simulink model "transfer_function_question_4_closed_loop"  (R2023b)
settings: Solver=VariableStepAuto  StartTime=0.0  StopTime=40  RelTol=1e-3
settings Model: Creator=orife  LastModifiedBy=orife

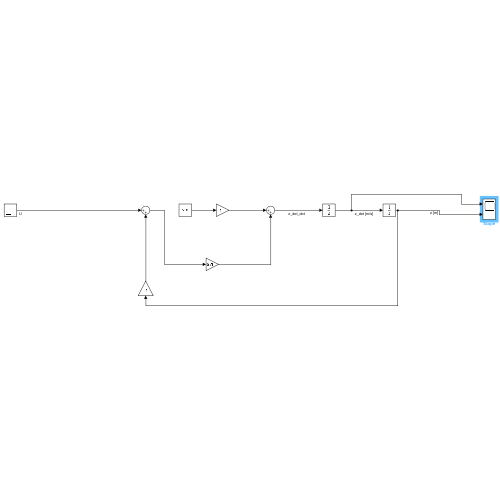
[thumbnail: Simulink's stored preview of the top-level diagram]
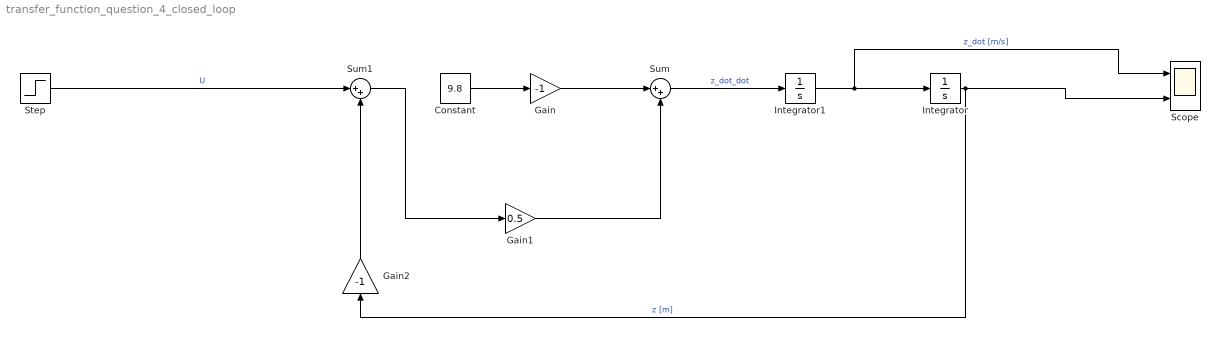
== system transfer_function_question_4_closed_loop ==
  Constant : Constant  Value=9.8
  Gain : Gain  Gain=-1
  Gain1 : Gain  Gain=0.5
  Gain2 : Gain  Gain=-1
  Integrator : Integrator  InitialCondition=5
  Integrator1 : Integrator
  Scope : Scope  NumInputPorts=2
  Step : Step  After=19.6  SampleTime=0
  Sum : Sum  Inputs=|++
  Sum1 : Sum  Inputs=|++
  wires:
  Integrator1/1 -> Scope/1, Integrator/1  "z_dot [m/s]"
  Constant/1 -> Gain/1
  Gain/1 -> Sum/1
  Sum/1 -> Integrator1/1  "z_dot_dot"
  Integrator/1 -> Gain2/1, Scope/2  "z [m]"
  Gain1/1 -> Sum/2
  Step/1 -> Sum1/1  "U"
  Sum1/1 -> Gain1/1
  Gain2/1 -> Sum1/2
